simulink library "INT_InjCrv_PoI2AddCor"  (R2016b)
settings: Solver=VariableStepAuto  StartTime=0.0  StopTime=10.0  RelTol=1e-3
settings Model: Creator=Administrator  LastModifiedBy=Administrator

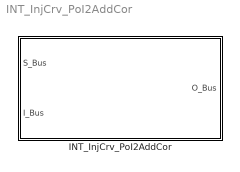
== system INT_InjCrv_PoI2AddCor ==
  INT_InjCrv_PoI2AddCor : Subsystem

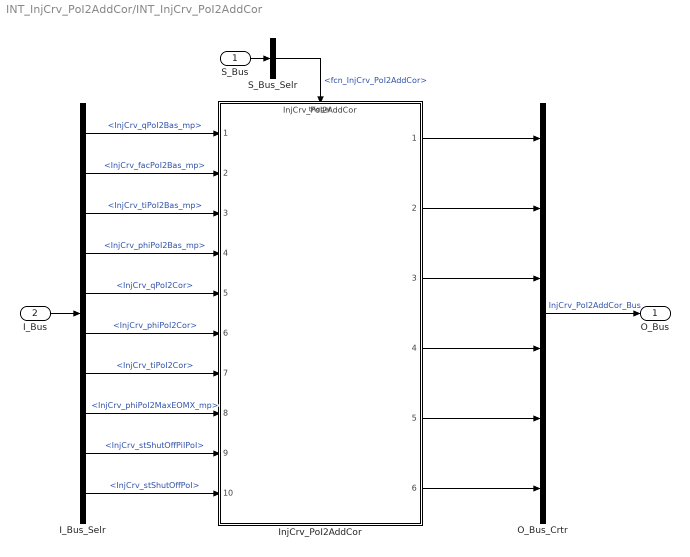
== system INT_InjCrv_PoI2AddCor/INT_InjCrv_PoI2AddCor ==
  S_Bus : Inport
  I_Bus : Inport  Port=2
  I_Bus_Selr : BusSelector  OutputSignals=InjCrv_qPoI2Bas_mp,InjCrv_facPoI2Bas_mp,InjCrv_tiPoI2Bas_mp,InjCrv_phiPoI2Bas_mp,InjCrv_qPoI2Cor,InjCrv_phiPoI2Cor,InjCrv_tiPoI2Cor,InjCrv_phiPoI2MaxEOMX_mp,InjCrv_stShutOffPiIPoI,InjCrv_stShutOffPoI
  InjCrv_PoI2AddCor : ModelReference  ModelNameDialog=InjCrv_PoI2AddCor  SimulationMode=Normal  ModelReferenceVersion=1.19  TriggerPortName=function  TriggerPortTriggerType=function-call  TriggerPortStatesWhenEnabling=held
  O_Bus_Crtr : BusCreator  Inputs=6
  S_Bus_Selr : BusSelector  OutputSignals=fcn_InjCrv_PoI2AddCor
  O_Bus : Outport
  wires:
  S_Bus_Selr/1 -> InjCrv_PoI2AddCor/Trigger  "<fcn_InjCrv_PoI2AddCor>"
  S_Bus/1 -> S_Bus_Selr/1
  I_Bus/1 -> I_Bus_Selr/1
  I_Bus_Selr/1 -> InjCrv_PoI2AddCor/1  "<InjCrv_qPoI2Bas_mp>"
  I_Bus_Selr/2 -> InjCrv_PoI2AddCor/2  "<InjCrv_facPoI2Bas_mp>"
  I_Bus_Selr/3 -> InjCrv_PoI2AddCor/3  "<InjCrv_tiPoI2Bas_mp>"
  I_Bus_Selr/4 -> InjCrv_PoI2AddCor/4  "<InjCrv_phiPoI2Bas_mp>"
  I_Bus_Selr/5 -> InjCrv_PoI2AddCor/5  "<InjCrv_qPoI2Cor>"
  I_Bus_Selr/6 -> InjCrv_PoI2AddCor/6  "<InjCrv_phiPoI2Cor>"
  I_Bus_Selr/7 -> InjCrv_PoI2AddCor/7  "<InjCrv_tiPoI2Cor>"
  I_Bus_Selr/8 -> InjCrv_PoI2AddCor/8  "<InjCrv_phiPoI2MaxEOMX_mp>"
  I_Bus_Selr/9 -> InjCrv_PoI2AddCor/9  "<InjCrv_stShutOffPiIPoI>"
  I_Bus_Selr/10 -> InjCrv_PoI2AddCor/10  "<InjCrv_stShutOffPoI>"
  O_Bus_Crtr/1 -> O_Bus/1  "InjCrv_PoI2AddCor_Bus"
  InjCrv_PoI2AddCor/1 -> O_Bus_Crtr/1
  InjCrv_PoI2AddCor/2 -> O_Bus_Crtr/2
  InjCrv_PoI2AddCor/3 -> O_Bus_Crtr/3
  InjCrv_PoI2AddCor/4 -> O_Bus_Crtr/4
  InjCrv_PoI2AddCor/5 -> O_Bus_Crtr/5
  InjCrv_PoI2AddCor/6 -> O_Bus_Crtr/6
